simulink model "motor"  (R2018b)
settings: Solver=VariableStepAuto  StartTime=0.0  StopTime=Endtime  RelTol=1e-3
values from neighbouring files (symbols this model uses):
  D = 6.0e-5    (= 6e-05)    [motor_sim.m]    (also in plant_model_sim.m)
  Ji = 1.3e-3    (= 0.0013)    [motor_sim.m]    (also in plant_model_sim.m)
  Jm = 0.11e-3    (= 0.00011)    [motor_sim.m]    (also in plant_model_sim.m)
  Ke = 7.16e-2    (= 0.0716)    [motor_sim.m]    (also in plant_model_sim.m)
  Kt = 7.2e-2    (= 0.072)    [motor_sim.m]    (also in plant_model_sim.m)
  L = 0.2    [motor_sim.m]    (also in plant_model_sim.m)
  R = 5.7    [motor_sim.m]    (also in plant_model_sim.m)
  v_M = 24    [motor_sim.m]    (also in plant_model_sim.m)
settings Model: Creator=nharada  LastModifiedBy=nharada

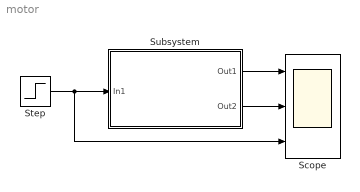
== system motor ==
  Scope : Scope  NumInputPorts=3
  Step : Step  After=v_M  SampleTime=0
  Subsystem : Subsystem
  wires:
  Step/1 -> Scope/3, Subsystem/1(In1)
  Subsystem/1(Out1) -> Scope/1
  Subsystem/2(Out2) -> Scope/2

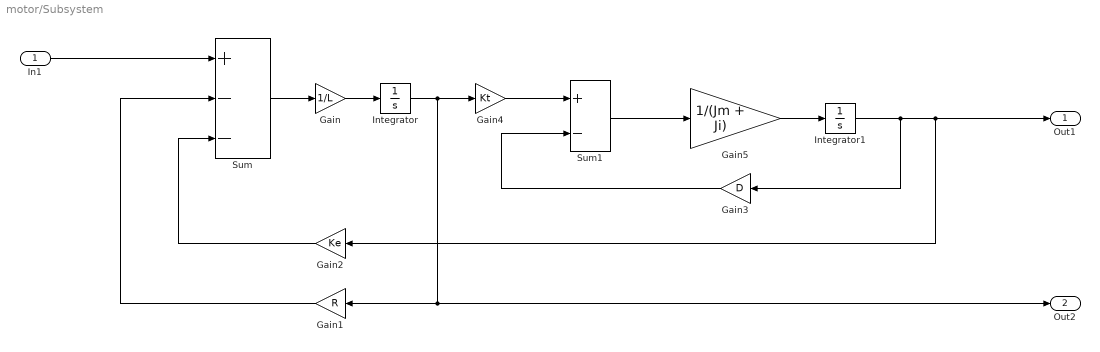
== system motor/Subsystem ==
  In1 : Inport
  Gain : Gain  Gain=1/L
  Gain1 : Gain  Gain=R
  Gain2 : Gain  Gain=Ke
  Gain3 : Gain  Gain=D
  Gain4 : Gain  Gain=Kt
  Gain5 : Gain  Gain=1/(Jm + Ji)
  Integrator : Integrator
  Integrator1 : Integrator
  Sum : Sum  Inputs=+--
  Sum1 : Sum  Inputs=+-
  Out1 : Outport
  Out2 : Outport  Port=2
  wires:
  Gain1/1 -> Sum/2
  Sum/1 -> Gain/1
  Gain3/1 -> Sum1/2
  Gain2/1 -> Sum/3
  Gain/1 -> Integrator/1
  Integrator1/1 -> Gain3/1, Out1/1, Gain2/1
  Integrator/1 -> Gain4/1, Out2/1, Gain1/1
  Sum1/1 -> Gain5/1
  Gain5/1 -> Integrator1/1
  Gain4/1 -> Sum1/1
  In1/1 -> Sum/1
